simulink model "afbs_control"  (R2015a)
settings: Solver=ode45  StartTime=0.0  StopTime=0.3  FixedStep=0.1  RelTol=1e-4
values from neighbouring files (symbols this model uses):
  sys = tf(sys_zpk)    [main.m]    (also in main_compare_single_dual.m; main_cost_space.m; myFitness.m; myFitness_lamba_u.m)
libraries: simulink x1
settings Model: Creator=Xiaotian  LastModifiedBy=Xiaotian

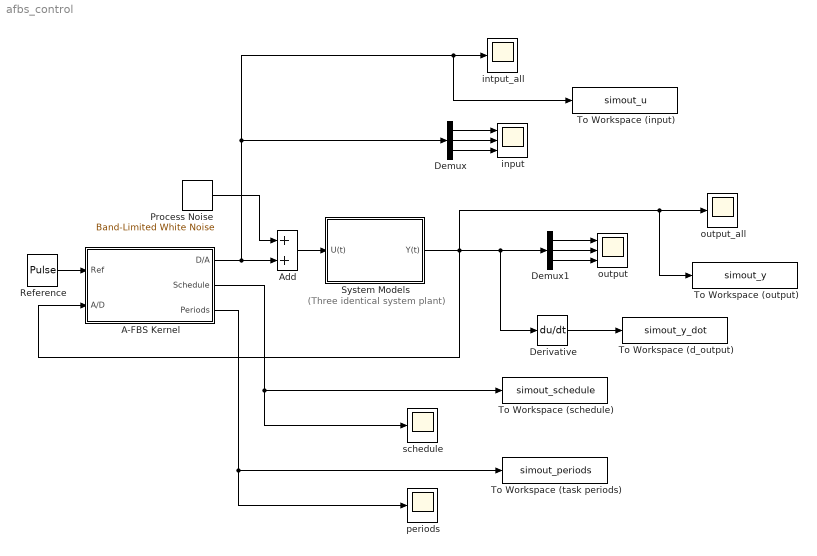
== system afbs_control ==
  note: (Three identical system plant)
  A-FBS Kernel : Subsystem  mask{Parameter=1}
  Add : Sum
  Demux : Demux  Outputs=3
  Demux1 : Demux  Outputs=3
  Derivative : Derivative
  Process Noise : simulink/Sources/Band-Limited White Noise  Cov=[0]  Ts=0.1  seed=[23341]
  Reference : DiscretePulseGenerator  PulseType=Time based  Period=1  PulseWidth=50
  System Models : Subsystem
  To Workspace (d_output) : ToWorkspace  VariableName=simout_y_dot  SaveFormat=Timeseries  SampleTime=-1
  To Workspace (input) : ToWorkspace  VariableName=simout_u  SaveFormat=Timeseries  SampleTime=-1
  To Workspace (output) : ToWorkspace  VariableName=simout_y  SaveFormat=Timeseries  SampleTime=-1
  To Workspace (schedule) : ToWorkspace  VariableName=simout_schedule  SaveFormat=Timeseries  SampleTime=-1
  To Workspace (task periods) : ToWorkspace  VariableName=simout_periods  SaveFormat=Timeseries  SampleTime=-1
  input : Scope  NumInputPorts=3
      settings: YMin=-5~-5~-5  YMax=5~5~5
  intput_all : Scope
      settings: SaveName=ScopeData4
  output : Scope  NumInputPorts=3
      settings: YMin=-5~-5~-5  YMax=5~5~5
  output_all : Scope
      settings: TimeRange=0.1  YMin=-0.6000000000000001  YMax=1.4  SaveName=ScopeData3
  periods : Scope
      settings: SaveName=ScopeData5
  schedule : Scope
      settings: SaveName=ScopeData2
  wires:
  A-FBS Kernel/2(Schedule) -> schedule/1, To Workspace (schedule)/1
  Demux1/3 -> output/3
  Demux1/2 -> output/2
  Demux1/1 -> output/1
  Demux/3 -> input/3
  Demux/2 -> input/2
  Demux/1 -> input/1
  A-FBS Kernel/3(Periods) -> periods/1, To Workspace (task periods)/1
  Reference/1 -> A-FBS Kernel/1(Ref)
  Derivative/1 -> To Workspace (d_output)/1
  Process Noise/1 -> Add/1
  Add/1 -> System Models/1(U(t))
  System Models/1(Y(t)) -> To Workspace (output)/1, output_all/1, Demux1/1, Derivative/1, A-FBS Kernel/2(A/D)
  A-FBS Kernel/1(D/A) -> Add/2, To Workspace (input)/1, intput_all/1, Demux/1

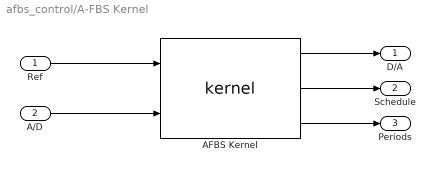
== system afbs_control/A-FBS Kernel ==
  Ref : Inport
  A/D : Inport  Port=2
  AFBS Kernel : S-Function  FunctionName=kernel  Parameters=alpha, h_h, h_l
  D/A : Outport
  Schedule : Outport  Port=2
  Periods : Outport  Port=3
  wires:
  AFBS Kernel/1 -> D/A/1
  AFBS Kernel/2 -> Schedule/1
  AFBS Kernel/3 -> Periods/1
  Ref/1 -> AFBS Kernel/1
  A/D/1 -> AFBS Kernel/2

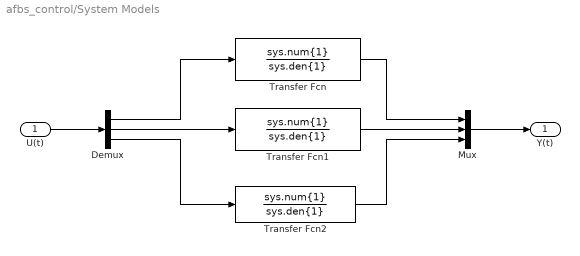
== system afbs_control/System Models ==
  U(t) : Inport
  Demux : Demux  Outputs=3
  Mux : Mux  Inputs=3
  Transfer Fcn : TransferFcn  Numerator=sys.num{1}  Denominator=sys.den{1}
  Transfer Fcn1 : TransferFcn  Numerator=sys.num{1}  Denominator=sys.den{1}
  Transfer Fcn2 : TransferFcn  Numerator=sys.num{1}  Denominator=sys.den{1}
  Y(t) : Outport
  wires:
  U(t)/1 -> Demux/1
  Demux/1 -> Transfer Fcn/1
  Demux/2 -> Transfer Fcn1/1
  Demux/3 -> Transfer Fcn2/1
  Transfer Fcn/1 -> Mux/1
  Transfer Fcn1/1 -> Mux/2
  Transfer Fcn2/1 -> Mux/3
  Mux/1 -> Y(t)/1
